simulink subsystem "euler_to_rw"  (R2022b)
settings: Solver=VariableStepAuto  StartTime=0.0  StopTime=10.0  RelTol=1e-3
settings Model: Creator=Jon  LastModifiedBy=Cal__
settings ModelReferenceCC: EnableRefExpFcnMdlSchedulingChecks=on

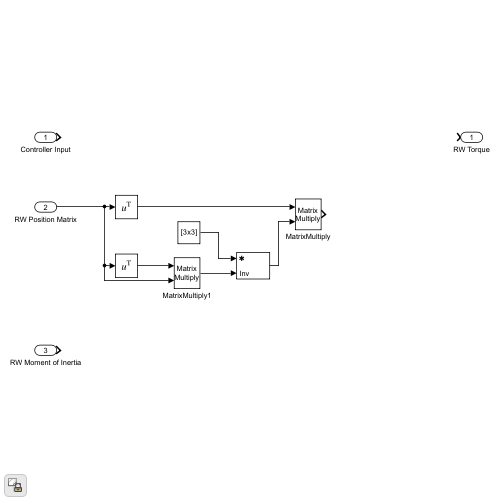
[thumbnail: Simulink's stored preview of the top-level diagram]
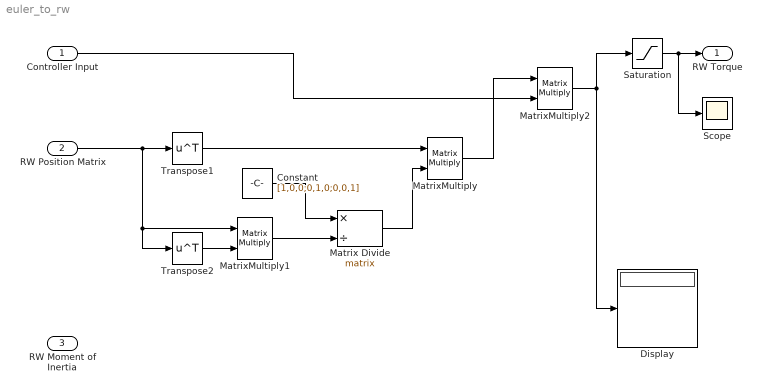
== system euler_to_rw ==
  Controller Input : Inport
  RW Position Matrix : Inport  Port=2
  RW Moment of Inertia : Inport  Port=3
  Constant : Constant  Value=[1,0,0;0,1,0;0,0,1]
  Display : Display
  Matrix Divide : Product  Inputs=*/  Multiplication=Matrix(*)
  MatrixMultiply : Product  Multiplication=Matrix(*)
  MatrixMultiply1 : Product  Multiplication=Matrix(*)
  MatrixMultiply2 : Product  Multiplication=Matrix(*)
  Saturation : Saturate  UpperLimit=55*10^-3  LowerLimit=-55*10^-3
  Scope : Scope
  Transpose1 : Math  Operator=transpose
  Transpose2 : Math  Operator=transpose
  RW Torque : Outport
  wires:
  RW Position Matrix/1 -> Transpose2/1, MatrixMultiply1/1, Transpose1/1
  Transpose2/1 -> MatrixMultiply1/2
  MatrixMultiply1/1 -> Matrix Divide/2
  Matrix Divide/1 -> MatrixMultiply/2
  Constant/1 -> Matrix Divide/1
  Transpose1/1 -> MatrixMultiply/1
  MatrixMultiply/1 -> MatrixMultiply2/1
  Controller Input/1 -> MatrixMultiply2/2
  MatrixMultiply2/1 -> Saturation/1, Display/1
  Saturation/1 -> RW Torque/1, Scope/1
